simulink model "topquantize"  (Simulink 6.3)
settings: Solver=FixedStepDiscrete  StartTime=0.0  StopTime=100  FixedStep=1  RelTol=1e-3
InitFcn:
  | %% DSPBuilder Start
  | alt_dspbuilder_update_model(bdroot)
  | %% DSPBuilder End
libraries: allblocks_alteradspbuilder2 x13, simulink x1
settings Model: LastModifiedBy=LKONG  StrictBusMsg=None
settings DataIOCC: SignalLoggingName=sigsOut
settings OptimizationCC: BooleanDataType=off  InlineInvariantSignals=on
settings DebuggingCC: SolverPrmCheckMsg=none
settings HardwareCC: TargetUnknown=on

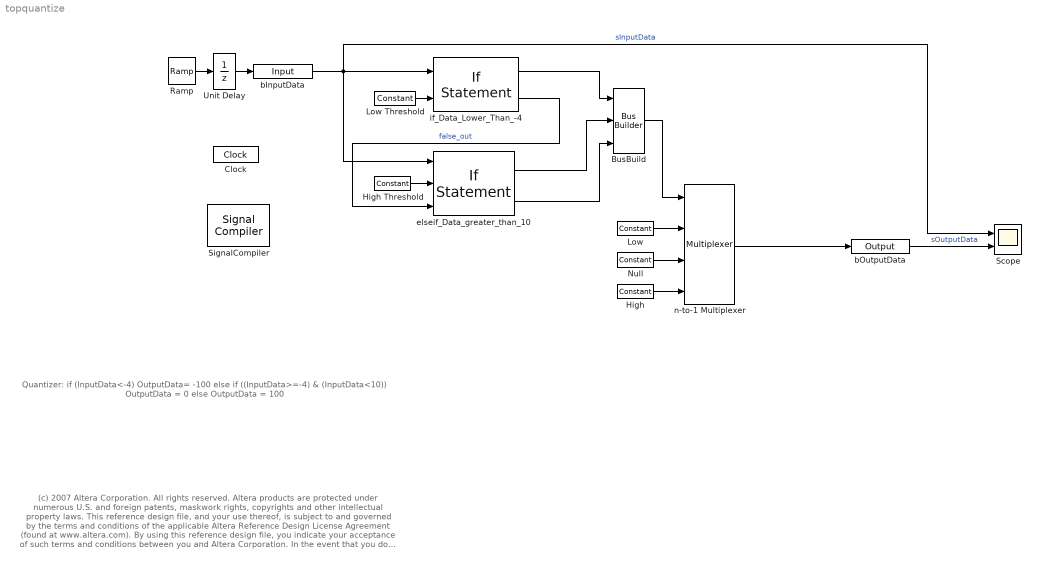
== system topquantize ==
  note: Quantizer:
      | if (InputData<-4)  OutputData= -100
      | else if ((InputData>=-4) & (InputData<10)) OutputData = 0
      | else OutputData = 100
  note: (c) 2007 Altera Corporation. All rights reserved.  Altera products are protected under numerous U.S. and foreign patents, maskwork rights, copyrights and other intellectual property laws.
      | This reference design file, and your use thereof, is subject to and governed by the terms and conditions of the applicable Altera Reference Design License Agreement (found at www.altera.com).
      | By using this reference design file, you indicate your acceptance of such terms and conditions between you and Altera Corporation.
      | In the event that you do not agree with such terms and conditions, you may not use the reference design file and please promptly destroy any copies you have made.
      | This reference design file being provided on an "as-is" basis and as an accommodation and therefore all warranties, representations or guarantees of any kind (whether express, implied or statutory)
      | including, without limitation, warranties of merchantability, non-infringement, or fitness for a particular purpose, are specifically disclaimed.
      | By making this reference design file available, Altera expressly does not recommend, suggest or require that this reference design file be used in combination with any other product not provided by Altera
  BusBuild : allblocks_alteradspbuilder2/Bus Builder  BusType=Unsigned Integer  bwl=3  bwr=0
  Clock : allblocks_alteradspbuilder2/Clock  ClockPeriod=100  ClockPeriodUnit=ns  SampleTime=1  SimulationStartCycle=5  PhaseOffset=0  Reset=aclr  ResetType=Active Low  Export=off
  High : allblocks_alteradspbuilder2/Constant  mask_cst=100  BusType=Signed Integer  bwl=8  bwr=0  SpecifyClock=off
  High Threshold : allblocks_alteradspbuilder2/Constant  mask_cst=10  BusType=Signed Integer  bwl=8  bwr=0  SpecifyClock=off
  Low : allblocks_alteradspbuilder2/Constant  mask_cst=-100  BusType=Signed Integer  bwl=8  bwr=0  SpecifyClock=off
  Low Threshold : allblocks_alteradspbuilder2/Constant  mask_cst=-4  BusType=Signed Integer  bwl=8  bwr=0  SpecifyClock=off
  Null : allblocks_alteradspbuilder2/Constant  mask_cst=0  BusType=Signed Integer  bwl=8  bwr=0  SpecifyClock=off
  Ramp : simulink/Sources/Ramp  slope=5  start=0  X0=0
  Scope : Scope  NumInputPorts=2
      settings: YMin=-5~-5  YMax=5~5
  SignalCompiler : allblocks_alteradspbuilder2/Signal Compiler  DeviceFamily=Stratix IV  DeviceName=AUTO  EnableSignalTap=off  SignalTapDepth=128  UseBoardBlock=off  StpUseDefaultClock=on  StpClock=Clock
  Unit Delay : UnitDelay
  bInputData : allblocks_alteradspbuilder2/Input  iofile=d:\wsTrunk\workspace\documentation\designExamples\demos\Transforms\Quantizer\tb_topquantize\topquantize_bInputData.salt  BusType=Signed Integer  bwl=8  bwr=0  SpecifyClock=off  PORTTYPE=Input
  bOutputData : allblocks_alteradspbuilder2/Output  iofile=d:\wsTrunk\workspace\documentation\designExamples\demos\Transforms\Quantizer\tb_topquantize\topquantize_bOutputData.capture  BusType=Signed Integer  bwl=8  bwr=0  PORTTYPE=Output
  elseif_Data_greater_than_10 : allblocks_alteradspbuilder2/If Statement  user_inputs=2  if_expression=a<b  BusType=Inferred  bwl=8  bwr=0  use_else_output=on  use_elseif_input=on
  if_Data_Lower_Than_-4 : allblocks_alteradspbuilder2/If Statement  user_inputs=2  if_expression=a<b  BusType=Inferred  bwl=8  bwr=0  use_else_output=on  use_elseif_input=off
  n-to-1 Multiplexer : allblocks_alteradspbuilder2/Multiplexer  numInputs=3  pipeline=0  oneHot=on  use_ena=off  use_aclr=off
  wires:
  Low Threshold/1 -> if_Data_Lower_Than_-4/2
  bInputData/1 -> if_Data_Lower_Than_-4/1, elseif_Data_greater_than_10/1, Scope/1  "sInputData"
  High Threshold/1 -> elseif_Data_greater_than_10/2
  Low/1 -> n-to-1 Multiplexer/2
  Null/1 -> n-to-1 Multiplexer/3
  High/1 -> n-to-1 Multiplexer/4
  n-to-1 Multiplexer/1 -> bOutputData/1
  Ramp/1 -> Unit Delay/1
  bOutputData/1 -> Scope/2  "sOutputData"
  BusBuild/1 -> n-to-1 Multiplexer/1
  if_Data_Lower_Than_-4/1 -> BusBuild/1
  elseif_Data_greater_than_10/1 -> BusBuild/2
  elseif_Data_greater_than_10/2 -> BusBuild/3
  if_Data_Lower_Than_-4/2 -> elseif_Data_greater_than_10/3  "false_out"
  Unit Delay/1 -> bInputData/1
